simulink model "gtcs_math_v0"  (R2022a)
settings: Solver=VariableStepAuto  StartTime=0.0  StopTime=28  RelTol=1e-3
values from neighbouring files (symbols this model uses):
  B_motor = 0.00025    [parameter_andar_servomotor.mat]    (also in parameter_original_servomotor.mat)
  J_motor = 0.0002548    [parameter_andar_servomotor.mat]    (also in parameter_original_servomotor.mat = 0.001)
  ke = 0.039313695    [parameter_andar_servomotor.mat]    (also in parameter_original_servomotor.mat = 0.04001501117)
  kt = 0.0378    [parameter_andar_servomotor.mat]    (also in parameter_original_servomotor.mat = 0.0375)
  L_motor = 6e-06    [parameter_andar_servomotor.mat]    (also in parameter_original_servomotor.mat = 3e-05)
  R_motor = 0.015    [parameter_andar_servomotor.mat]    (also in parameter_original_servomotor.mat = 0.075)
undefined symbols (not defined in the file or in its folder): sigbuilder_block
libraries: simulink x3
settings Model: Creator=yusuf.ogut  LastModifiedBy=yusuf.ogut

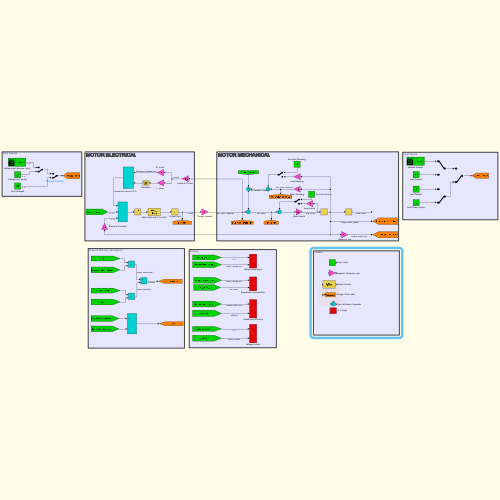
[thumbnail: Simulink's stored preview of the top-level diagram]
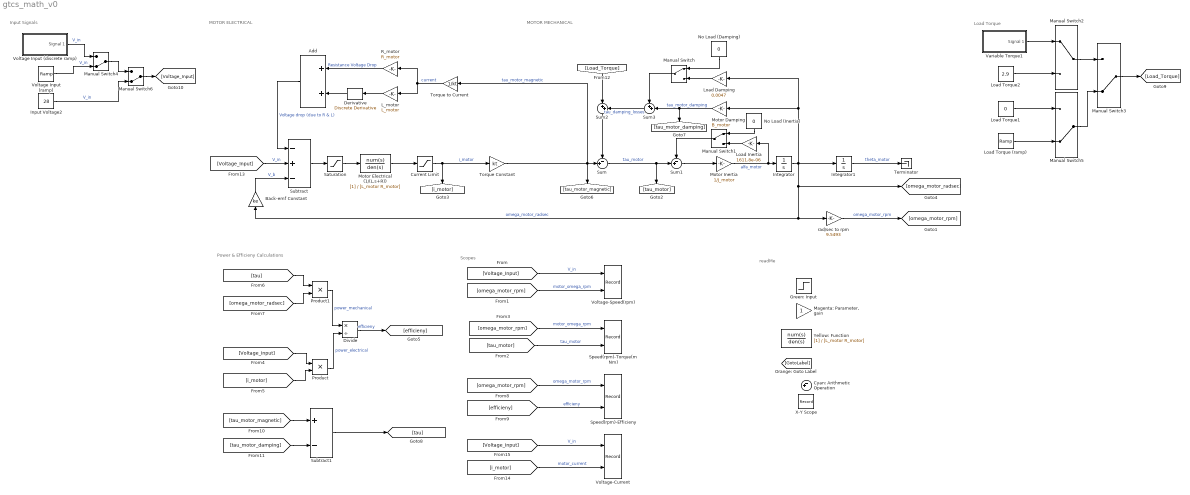
== system gtcs_math_v0 ==
  note: readMe
  note: MOTOR ELECTRICAL
  note: MOTOR MECHANICAL
  note: Load Torque
  note: Input Signals
  note: Scopes
  note: Power & Efficieny Calculations
  Add : Sum
  Back-emf Constant : Gain  Gain=ke
  Current Limit : Saturate  UpperLimit=80  LowerLimit=0
  Cyan: Arithmetic Operation : Sum  Inputs=-+|
  Derivative : simulink/Discrete/Discrete Derivative  gainval=1.0  ICPrevScaledInput=0.0  OutMin=[]  OutMax=[]  OutDataType=fixdt(1, 16)  OutScaling=2^-10  DoSatur=off
  Divide : Product  Inputs=*/
  Green: Input : Step  SampleTime=0
  Input Voltage2 : Constant  Value=28
  Integrator : Integrator
  Integrator1 : Integrator
  L_motor : Gain  Gain=L_motor
  Load Damping : Gain  Gain=0.0047
  Load Inertia : Gain  Gain=1611.8e-06
  Load Torque (ramp) : simulink/Sources/Ramp  slope=2.9/27  start=0  InitialOutput=1e-06
  Load Torque1 : Constant  Value=0
  Load Torque2 : Constant  Value=2.9
  "Magenta: Parameter, gain" : Gain
  Manual Switch : ManualSwitch
  Manual Switch1 : ManualSwitch
  Manual Switch2 : ManualSwitch
  Manual Switch{3..6} (4 alike) : ManualSwitch  CurrentSetting=0
  Motor Damping : Gain  Gain=B_motor
  Motor Electrical (1/(L.s+R)) : TransferFcn  Denominator=[L_motor R_motor]
  Motor Inertia : Gain  Gain=1/J_motor
  No Load (Damping) : Constant  Value=0
  No Load (Inertia) : Constant  Value=0
  Product : Product
  Product1 : Product
  R_motor : Gain  Gain=R_motor
  Saturation : Saturate  UpperLimit=28  LowerLimit=0
  Speed(rpm)-Efficieny : Record  FileSettingsInternal="{\"entries\":[{\"content\":{\"excelSettings\":{\"content\":{},\"type\":\"Streamout.ExcelSettings\"}},\"type\":\"Streamout.FileSettingStorage\",\"uuid\":\"7df471fc-6218-412d-9226-816465d27147\"}],\"packageUris\":[\"http://schema.mathworks.com/mf0/streamout_blocks/R2020a\"],\"version\":\"1.0\"}"  Layout=[1 1]  SignalsInternal="{\"entries\":[{\"content\":{\"signals\":[{\"content\":{\"blockPath\":[\"deneme_4/Speed(rpm)-Efficieny\"],\"channel\":[],\"dimensions\":[1],\"domain\":\"deneme_4/Speed(rpm)-Efficieny\",\"lineColor\":\"#d95319\",\"plots\":[1],\"port\":1,\"sid\":[\"\"],\"signalID\":19411,\"signalName\":\"omega_motor_rpm\"},\"type\":\"RecordBlkView.Signal\",\"uuid\":\"8fa2ed62-4937-47c5-90d1-dc8a64c4ba1a\"},{\"content\":{\"blockPath\":[\"deneme_4/Speed(rpm)-Efficieny\"],\"channel\":[],\"dimensions\":[1],\"domain\":\"deneme_4/Speed(rpm)-Efficieny\",\"lineColor\":\"#edb120\",\"plots\":[1],\"port\":2,\"sid\":[\"\"],\"signalID\":19415,\"signalName\":\"efficieny\"},\"type\":\"RecordBlkView.Signal\",\"uuid\":\"42833f9c-2654-4f2b-9d12-de49e0719e9a\"}]},\"type\":\"RecordBlkView.InputSignals\",\"uuid\":\"b2a9eec3-c8c3-495c-affc-ed6feddd1ffc\"}],\"packageUris\":[\"http://schema.mathworks.com/mf0/streamout_blocks/R2020a\"],\"version\":\"1.0\"}"  VisualizationBindings="{\"xyplotplugin\":{\"info\":[{\"series\":[{\"bindingParametersList\":[{\"parameter\":\"X-Axis\",\"signalID\":19411,\"signalName\":\"omega_motor_rpm\"},{\"parameter\":\"Y-Axis\",\"signalID\":19415,\"signalName\":\"efficieny\"}],\"seriesID\":26403}],\"subplotID\":1}]}}"  CompatibilityTag=XY
  Speed(rpm)-Torque(mNm) : Record  FileSettingsInternal="{\"entries\":[{\"content\":{\"excelSettings\":{\"content\":{},\"type\":\"Streamout.ExcelSettings\"}},\"type\":\"Streamout.FileSettingStorage\",\"uuid\":\"315ed191-27cf-4af2-b047-4df13758ca00\"}],\"packageUris\":[\"http://schema.mathworks.com/mf0/streamout_blocks/R2020a\"],\"version\":\"1.0\"}"  Layout=[1 1]  SignalsInternal="{\"entries\":[{\"content\":{\"signals\":[{\"content\":{\"blockPath\":[\"deneme_4/Speed(rpm)-Torque(mNm)\"],\"channel\":[],\"dimensions\":[1],\"domain\":\"deneme_4/Speed(rpm)-Torque(mNm)\",\"lineColor\":\"#7e2f8e\",\"plots\":[1],\"port\":1,\"sid\":[\"\"],\"signalID\":19419,\"signalName\":\"motor_omega_rpm\"},\"type\":\"RecordBlkView.Signal\",\"uuid\":\"573bfe5e-4eaa-404f-9fbe-c5071d5e986b\"},{\"content\":{\"blockPath\":[\"deneme_4/Speed(rpm)-Torque(mNm)\"],\"channel\":[],\"dimensions\":[1],\"domain\":\"deneme_4/Speed(rpm)-Torque(mNm)\",\"lineColor\":\"#77ac30\",\"plots\":[1],\"port\":2,\"sid\":[\"\"],\"signalID\":19423,\"signalName\":\"tau_motor\"},\"type\":\"RecordBlkView.Signal\",\"uuid\":\"e6281e5d-d311-4ca1-a728-1e6e06521eb3\"}]},\"type\":\"RecordBlkView.InputSignals\",\"uuid\":\"0769ebf3-4200-4932-8038-1bf2905a68f6\"}],\"packageUris\":[\"http://schema.mathworks.com/mf0/streamout_blocks/R2020a\"],\"version\":\"1.0\"}"  VisualizationBindings="{\"xyplotplugin\":{\"info\":[{\"series\":[{\"bindingParametersList\":[{\"parameter\":\"X-Axis\",\"signalID\":19419,\"signalName\":\"motor_omega_rpm\"},{\"parameter\":\"Y-Axis\",\"signalID\":19423,\"signalName\":\"tau_motor\"}],\"seriesID\":48988}],\"subplotID\":1}]}}"  CompatibilityTag=XY
  Subtract : Sum  Inputs=-+-
  Subtract1 : Sum  Inputs=+-
  Sum : Sum  Inputs=-+|
  Sum1 : Sum  Inputs=-+|
  Sum2 : Sum  Inputs=|++
  Sum3 : Sum  Inputs=++|
  Terminator : Terminator
  Torque Constant : Gain  Gain=kt
  Torque to Current : Gain  Gain=1/kt
  Variable Torque1 : Subsystem  Tag=STV Subsys  LoadFcn=sigbuilder_block('load');  StartFcn=sigbuilder_block('start');  StopFcn=sigbuilder_block('stop');  ClipboardFcn=sigbuilder_block('clipboard');  mask(Sigbuilder block){tuvar=[0:10]}
      mask help: Simulink:masks:SigbuilderBlock_MD
      mask init:
      | if ~strcmp(get_param(bdroot(gcbh),'SimulationStatus'),'stopped') tuvar = sigbuilder_block('maskInit'); end
      settings: CopyFcn=sigbuilder_block('copy');  DeleteFcn=sigbuilder_block('delete');  ModelCloseFcn=sigbuilder_block('modelClose');  PreSaveFcn=sigbuilder_block('preSave');  PauseFcn=sigbuilder_block('pause');  ContinueFcn=sigbuilder_block('continue');  NameChangeFcn=sigbuilder_block('namechange');  OpenFcn=sigbuilder_block('open',[0 36 1440 716.25 ]);  CloseFcn=sigbuilder_block('close');
      mask Display: plot(0, 0, 100, 100,[2, 2, 32, 32, 2], [68, 8, 8, 68, 68],[32, 2], [38, 38], [32, 19, 2],[53, 60, 44], [32, 17, 17, 2],[16, 16, 31, 31]);txt = getActiveGroup(gcbh);text(2, 100, txt,'verticalAlignment', 'top');
  Voltage Input (discrete ramp) : Subsystem  Tag=STV Subsys  LoadFcn=sigbuilder_block('load');  StartFcn=sigbuilder_block('start');  StopFcn=sigbuilder_block('stop');  ClipboardFcn=sigbuilder_block('clipboard');  mask(Sigbuilder block){tuvar=[0:10]}
      mask help: Simulink:masks:SigbuilderBlock_MD
      mask init:
      | if ~strcmp(get_param(bdroot(gcbh),'SimulationStatus'),'stopped') tuvar = sigbuilder_block('maskInit'); end
      settings: CopyFcn=sigbuilder_block('copy');  DeleteFcn=sigbuilder_block('delete');  ModelCloseFcn=sigbuilder_block('modelClose');  PreSaveFcn=sigbuilder_block('preSave');  PauseFcn=sigbuilder_block('pause');  ContinueFcn=sigbuilder_block('continue');  NameChangeFcn=sigbuilder_block('namechange');  OpenFcn=sigbuilder_block('open',[0.75 36.75 718.5 709.5 ]);  CloseFcn=sigbuilder_block('close');
      mask Display: plot(0, 0, 100, 100,[2, 2, 32, 32, 2], [68, 8, 8, 68, 68],[32, 2], [38, 38], [32, 19, 2],[53, 60, 44], [32, 17, 17, 2],[16, 16, 31, 31]);txt = getActiveGroup(gcbh);text(2, 100, txt,'verticalAlignment', 'top');
  Voltage Input (ramp) : simulink/Sources/Ramp  slope=28/28  start=0  InitialOutput=0
  Voltage-Current : Record  FileSettingsInternal="{\"entries\":[{\"content\":{\"excelSettings\":{\"content\":{},\"type\":\"Streamout.ExcelSettings\"}},\"type\":\"Streamout.FileSettingStorage\",\"uuid\":\"9deadd68-2624-47f6-bc80-4eec0aa71c1f\"}],\"packageUris\":[\"http://schema.mathworks.com/mf0/streamout_blocks/R2020a\"],\"version\":\"1.0\"}"  Layout=[1 1]  SignalsInternal="{\"entries\":[{\"content\":{\"signals\":[{\"content\":{\"blockPath\":[\"deneme_4/Voltage-Current\"],\"channel\":[],\"dimensions\":[1],\"domain\":\"deneme_4/Voltage-Current\",\"lineColor\":\"#ff13a6\",\"plots\":[1],\"port\":1,\"sid\":[\"\"],\"signalID\":19483,\"signalName\":\"V_in\"},\"type\":\"RecordBlkView.Signal\",\"uuid\":\"c032b403-6174-433b-8861-fdb8f2881ace\"},{\"content\":{\"blockPath\":[\"deneme_4/Voltage-Current\"],\"channel\":[],\"dimensions\":[1],\"domain\":\"deneme_4/Voltage-Current\",\"lineColor\":\"#fe330a\",\"plots\":[1],\"port\":2,\"sid\":[\"\"],\"signalID\":19487,\"signalName\":\"motor_current\"},\"type\":\"RecordBlkView.Signal\",\"uuid\":\"9bcaccaa-3ce8-4d5b-8330-37171a30f83a\"}]},\"type\":\"RecordBlkView.InputSignals\",\"uuid\":\"4a1af164-b1be-44ad-af18-d57e7ad29d3a\"}],\"packageUris\":[\"http://schema.mathworks.com/mf0/streamout_blocks/R2020a\"],\"version\":\"1.0\"}"  VisualizationBindings="{\"xyplotplugin\":{\"info\":[{\"series\":[{\"bindingParametersList\":[{\"parameter\":\"X-Axis\",\"signalID\":19483,\"signalName\":\"V_in\"},{\"parameter\":\"Y-Axis\",\"signalID\":19487,\"signalName\":\"motor_current\"}],\"seriesID\":1906}],\"subplotID\":1}]}}"  CompatibilityTag=XY
  Voltage-Speed(rpm) : Record  FileSettingsInternal="{\"entries\":[{\"content\":{\"excelSettings\":{\"content\":{},\"type\":\"Streamout.ExcelSettings\"}},\"type\":\"Streamout.FileSettingStorage\",\"uuid\":\"21ada231-7678-4e9f-96f9-58e67c5ec8dc\"}],\"packageUris\":[\"http://schema.mathworks.com/mf0/streamout_blocks/R2020a\"],\"version\":\"1.0\"}"  Layout=[1 1]  SignalsInternal="{\"entries\":[{\"content\":{\"signals\":[{\"content\":{\"blockPath\":[\"deneme_4/Voltage-Speed(rpm)\"],\"channel\":[],\"dimensions\":[1],\"domain\":\"deneme_4/Voltage-Speed(rpm)\",\"lineColor\":\"#7e2f8e\",\"plots\":[1],\"port\":1,\"sid\":[\"\"],\"signalID\":19491,\"signalName\":\"V_in\"},\"type\":\"RecordBlkView.Signal\",\"uuid\":\"6a28d7d5-b34d-4bb4-90cb-0c0761e3f10c\"},{\"content\":{\"blockPath\":[\"deneme_4/Voltage-Speed(rpm)\"],\"channel\":[],\"dimensions\":[1],\"domain\":\"deneme_4/Voltage-Speed(rpm)\",\"lineColor\":\"#d95319\",\"plots\":[1],\"port\":2,\"sid\":[\"\"],\"signalID\":19495,\"signalName\":\"motor_omega_rpm\"},\"type\":\"RecordBlkView.Signal\",\"uuid\":\"addf5390-c670-4d39-acb8-3a0623c1176b\"}]},\"type\":\"RecordBlkView.InputSignals\",\"uuid\":\"3b794c6d-c6fd-4a08-8164-6460a5de0d51\"}],\"packageUris\":[\"http://schema.mathworks.com/mf0/streamout_blocks/R2020a\"],\"version\":\"1.0\"}"  VisualizationBindings="{\"xyplotplugin\":{\"info\":[{\"series\":[{\"bindingParametersList\":[{\"parameter\":\"X-Axis\",\"signalID\":19491,\"signalName\":\"V_in\"},{\"parameter\":\"Y-Axis\",\"signalID\":19495,\"signalName\":\"motor_omega_rpm\"}],\"seriesID\":30810}],\"subplotID\":1}]}}"  CompatibilityTag=XY
  X-Y Scope : Record  FileSettingsInternal="{\"entries\":[{\"content\":{\"excelSettings\":{\"content\":{},\"type\":\"Streamout.ExcelSettings\"}},\"type\":\"Streamout.FileSettingStorage\",\"uuid\":\"0f904335-7ad7-4e23-8479-2fe4c462a63c\"}],\"packageUris\":[\"http://schema.mathworks.com/mf0/streamout_blocks/R2020a\"],\"version\":\"1.0\"}"  Layout=[1 1]  SignalsInternal="{\"entries\":[{\"content\":{\"signals\":[{\"content\":{\"blockPath\":[\"deneme_4/X-Y Scope\"],\"channel\":[],\"dimensions\":[1],\"domain\":\"deneme_4/X-Y Scope\",\"lineColor\":\"#fe330a\",\"plots\":[],\"port\":1,\"sid\":[\"\"],\"signalID\":19511},\"type\":\"RecordBlkView.Signal\",\"uuid\":\"0ff1d7dc-f8e1-49ae-a194-e317b15a0efa\"},{\"content\":{\"blockPath\":[\"deneme_4/X-Y Scope\"],\"channel\":[],\"dimensions\":[1],\"domain\":\"deneme_4/X-Y Scope\",\"lineColor\":\"#22b573\",\"plots\":[],\"port\":2,\"sid\":[\"\"],\"signalID\":19515},\"type\":\"RecordBlkView.Signal\",\"uuid\":\"bde43993-763d-4637-807e-0a4c3cd73386\"}]},\"type\":\"RecordBlkView.InputSignals\",\"uuid\":\"473bef71-7724-4e79-95b4-65485aa9b7b2\"}],\"packageUris\":[\"http://schema.mathworks.com/mf0/streamout_blocks/R2020a\"],\"version\":\"1.0\"}"  VisualizationBindings="{\"xyplotplugin\":{\"info\":[{\"series\":[],\"subplotID\":1}]}}"  CompatibilityTag=XY
  Yellow: Function : TransferFcn  Denominator=[L_motor R_motor]
  rad/sec to rpm : Gain  Gain=9.5493
  wires:
  Subtract/1 -> Saturation/1
  Torque Constant/1 -> Sum/2, [tau_motor_magnetic], Torque to Current/1  "tau_motor_magnetic"
  Motor Inertia/1 -> Load Inertia/1, Integrator/1  "alfa_motor"
  Integrator/1 -> rad/sec to rpm/1, Back-emf Constant/1, [omega_motor_radsec], Integrator1/1, Load Damping/1, Motor Damping/1  "omega_motor_radsec"
  Back-emf Constant/1 -> Subtract/3  "V_b"
  Integrator1/1 -> Terminator/1  "theta_motor"
  rad/sec to rpm/1 -> [omega_motor_rpm]  "omega_motor_rpm"
  Motor Electrical (1/(L.s+R))/1 -> Current Limit/1
  [Voltage_Input] -> Subtract/2  "V_in"
  [Voltage_Input] -> Voltage-Speed(rpm)/1  "V_in"
  [omega_motor_rpm] -> Voltage-Speed(rpm)/2  "motor_omega_rpm"
  [omega_motor_rpm] -> Speed(rpm)-Torque(mNm)/1  "motor_omega_rpm"
  [tau_motor] -> Speed(rpm)-Torque(mNm)/2  "tau_motor"
  [omega_motor_rpm] -> Speed(rpm)-Efficieny/1  "omega_motor_rpm"
  [efficieny] -> Speed(rpm)-Efficieny/2  "efficieny"
  Product1/1 -> Divide/1  "power_mechanical"
  Product/1 -> Divide/2  "power_electrical"
  [i_motor] -> Product/2
  [omega_motor_radsec] -> Product1/2
  [tau] -> Product1/1
  Divide/1 -> [efficieny]  "efficieny"
  [Voltage_Input] -> Product/1
  Current Limit/1 -> Torque Constant/1, [i_motor]  "i_motor"
  Saturation/1 -> Motor Electrical (1/(L.s+R))/1
  Motor Damping/1 -> Sum3/2, [tau_motor_damping]  "tau_motor_damping"
  Sum1/1 -> Motor Inertia/1
  Sum/1 -> Sum1/2, [tau_motor]  "tau_motor"
  L_motor/1 -> Derivative/1
  Torque to Current/1 -> R_motor/1, L_motor/1  "current"
  Derivative/1 -> Add/2
  R_motor/1 -> Add/1  "Resistance Voltage Drop"
  Add/1 -> Subtract/1  "Voltage drop (due to R & L)"
  Sum2/1 -> Sum/1
  [Load_Torque] -> Sum2/1
  [tau_motor_magnetic] -> Subtract1/1
  [tau_motor_damping] -> Subtract1/2
  Subtract1/1 -> [tau]
  Load Damping/1 -> Manual Switch/2
  No Load (Damping)/1 -> Manual Switch/1
  Load Inertia/1 -> Manual Switch1/2
  No Load (Inertia)/1 -> Manual Switch1/1
  Manual Switch1/1 -> Sum1/1
  Variable Torque1/1(Signal 1) -> Manual Switch2/1
  Load Torque2/1 -> Manual Switch2/2
  Manual Switch2/1 -> Manual Switch3/1
  Manual Switch3/1 -> [Load_Torque]
  Voltage Input (discrete ramp)/1(Signal 1) -> Manual Switch4/1  "V_in"
  Voltage Input (ramp)/1 -> Manual Switch4/2  "V_in"
  Input Voltage2/1 -> Manual Switch6/2  "V_in"
  Manual Switch4/1 -> Manual Switch6/1
  Manual Switch6/1 -> [Voltage_Input]
  Manual Switch/1 -> Sum3/1
  Sum3/1 -> Sum2/2  "tau_damping_losses"
  Load Torque (ramp)/1 -> Manual Switch5/2
  Load Torque1/1 -> Manual Switch5/1
  Manual Switch5/1 -> Manual Switch3/2
  [Voltage_Input] -> Voltage-Current/1  "V_in"
  [i_motor] -> Voltage-Current/2  "motor_current"

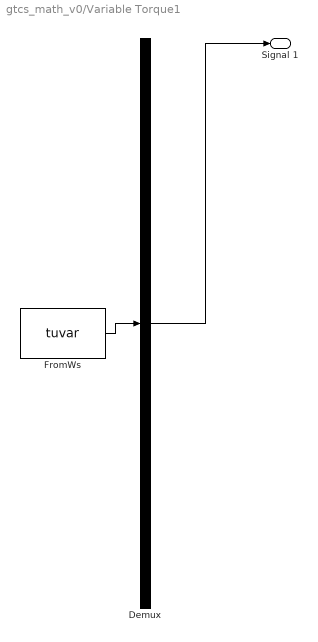
== system gtcs_math_v0/Variable Torque1 ==
  Demux : Demux  Tag=STV Demux  Outputs=1
      settings: DisplayOption=none
  FromWs : FromWorkspace  Tag=STV FromWs  VariableName=tuvar
      SigBuilderData=|
      | common.afterFinalStr = 'Extrapolate'
      | common.sampleTime = 0
      | dataSet.timeRange = [0 30]
      | dataSet.name = 'Group 1'
      | sbobj.Groups.Name = 'Group 1'
      | sbobj.Groups.Signals.Name = 'Signal 1'
      | sbobj.Groups.Signals.XData = [0 2 2 6 6 10 10 15 15 30]
      | sbobj.Groups.Signals.YData = [0 0 1 1 2 2 2.5 2.5 3 3]
      | sbobj.Groups.TimeRange = [0 30]
  Signal 1 : Outport  Tag=STV Outport
  wires:
  Demux/1 -> Signal 1/1
  FromWs/1 -> Demux/1

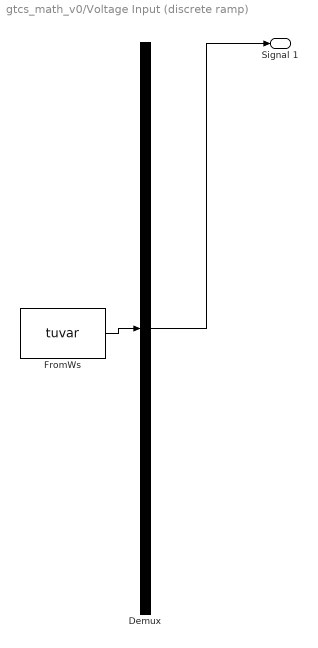
== system gtcs_math_v0/Voltage Input (discrete ramp) ==
  Demux : Demux  Tag=STV Demux  Outputs=1
      settings: DisplayOption=none
  FromWs : FromWorkspace  Tag=STV FromWs  VariableName=tuvar
      SigBuilderData=|
      | common.afterFinalStr = 'Extrapolate'
      | common.sampleTime = 0
      | dataSet.timeRange = [0 34]
      | dataSet.name = 'Group 1'
      | sbobj.Groups.Name = 'Group 1'
      | sbobj.Groups.Signals.Name = 'Signal 1'
      | sbobj.Groups.Signals.XData = [0 8 10 12 14 16 18 20 22 24 26 28 30 32 34]
      | sbobj.Groups.Signals.YData = [0 3.27 3.27 7.28 7.28 11.23 11.23 15.19 15.19 19.17 19.17 23.18 23.18 32 32]
      | sbobj.Groups.TimeRange = [0 34]
  Signal 1 : Outport  Tag=STV Outport
  wires:
  FromWs/1 -> Demux/1
  Demux/1 -> Signal 1/1
